simulink model "inv_pend_delay"  (Simulink 8.6)
settings: Solver=ode45  StartTime=0.0  StopTime=25  RelTol=1e-3
settings Model: Creator=mengg_000  LastModifiedBy=Gabriel
settings DebuggingCC: FcnCallInpInsideContextMsg=UseLocalSettings

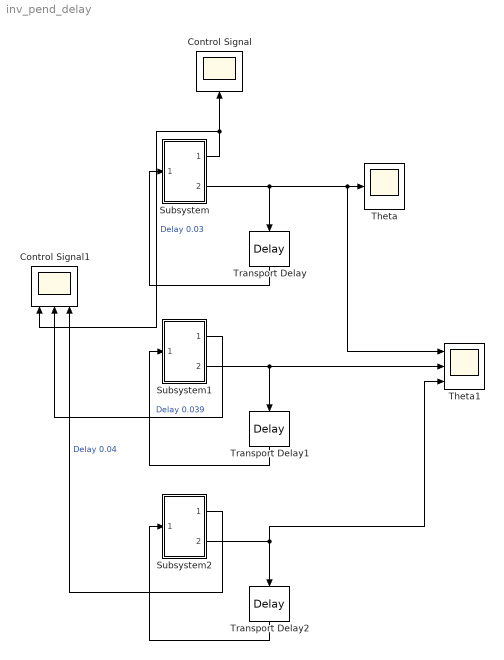
== system inv_pend_delay ==
  Control Signal : Scope
  Control Signal1 : Scope  NumInputPorts=3
  Subsystem : Subsystem
  Subsystem1 : Subsystem
  Subsystem2 : Subsystem
  Theta : Scope
  Theta1 : Scope  NumInputPorts=3
  Transport Delay : TransportDelay  DelayTime=0.03
  Transport Delay1 : TransportDelay  DelayTime=0.039
  Transport Delay2 : TransportDelay  DelayTime=0.04
  wires:
  Subsystem/2(Out2) -> Theta1/1, Theta/1, Transport Delay/1
  Transport Delay/1 -> Subsystem/1(In1)
  Subsystem/1(Out1) -> Control Signal1/1, Control Signal/1  "Delay 0.03"
  Subsystem1/2(Out2) -> Theta1/2, Transport Delay1/1
  Transport Delay1/1 -> Subsystem1/1(In1)
  Subsystem2/2(Out2) -> Theta1/3, Transport Delay2/1
  Transport Delay2/1 -> Subsystem2/1(In1)
  Subsystem1/1(Out1) -> Control Signal1/2  "Delay 0.039"
  Subsystem2/1(Out1) -> Control Signal1/3  "Delay 0.04"

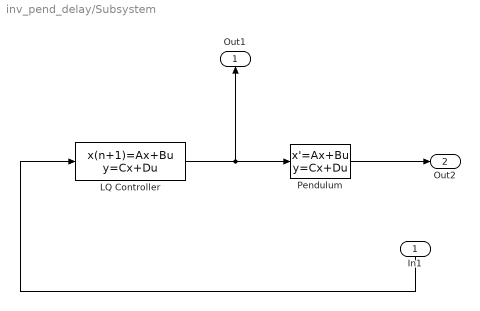
== system inv_pend_delay/Subsystem ==
  In1 : Inport
  LQ Controller : DiscreteStateSpace  A=|  B=|  C="[-12.1798  -13.3262         0]"  D=-8.1263  X0="[0;    0;   0]"  SampleTime=0.02
      A=|
      | [0.0389   -1.5001         0;
      |     0.0828    0.3594         0;
      |   -12.1798  -13.3262         0]
      B=|
      | [ -0.4344;
      |     0.1355;
      |    -8.1263]
  "Pendulum " : StateSpace  A=[0 3.0628;32 0]  B=[2; 0]  C=[0 1.5314]  D=0  X0=[0; 0.1]
  Out1 : Outport
  Out2 : Outport  Port=2
  wires:
  "Pendulum "/1 -> Out2/1
  In1/1 -> LQ Controller/1
  LQ Controller/1 -> Out1/1, "Pendulum "/1

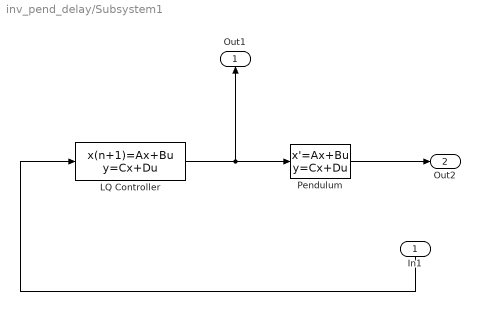
== system inv_pend_delay/Subsystem1 ==
  In1 : Inport
  LQ Controller : DiscreteStateSpace  A=|  B=|  C="[-12.1798  -13.3262         0]"  D=-8.1263  X0="[0;    0;   0]"  SampleTime=0.02
      A=|
      | [0.0389   -1.5001         0;
      |     0.0828    0.3594         0;
      |   -12.1798  -13.3262         0]
      B=|
      | [ -0.4344;
      |     0.1355;
      |    -8.1263]
  "Pendulum " : StateSpace  A=[0 3.0628;32 0]  B=[2; 0]  C=[0 1.5314]  D=0  X0=[0; 0.1]
  Out1 : Outport
  Out2 : Outport  Port=2
  wires:
  LQ Controller/1 -> "Pendulum "/1, Out1/1
  In1/1 -> LQ Controller/1
  "Pendulum "/1 -> Out2/1

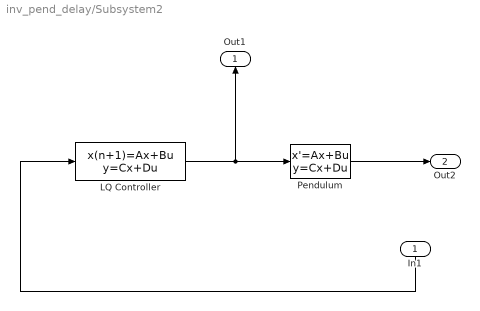
== system inv_pend_delay/Subsystem2 ==
  In1 : Inport
  LQ Controller : DiscreteStateSpace  A=|  B=|  C="[-12.1798  -13.3262         0]"  D=-8.1263  X0="[0;    0;   0]"  SampleTime=0.02
      A=|
      | [0.0389   -1.5001         0;
      |     0.0828    0.3594         0;
      |   -12.1798  -13.3262         0]
      B=|
      | [ -0.4344;
      |     0.1355;
      |    -8.1263]
  "Pendulum " : StateSpace  A=[0 3.0628;32 0]  B=[2; 0]  C=[0 1.5314]  D=0  X0=[0; 0.1]
  Out1 : Outport
  Out2 : Outport  Port=2
  wires:
  "Pendulum "/1 -> Out2/1
  In1/1 -> LQ Controller/1
  LQ Controller/1 -> Out1/1, "Pendulum "/1
